simulink model "verify_Pressure_Drop_Ceta_mdl"  (R2016b)
settings: Solver=VariableStepDiscrete  StartTime=0.0  StopTime=100  MaxStep=10  RelTol=1e-3  EnableMultiTasking=on
libraries: carnot x3, simulink x1
settings Model: Creator=drhf  LastModifiedBy=drhf
settings DataIOCC: LimitDataPoints=on  SaveFormat=Array  SignalLoggingSaveFormat=ModelDataLogs
settings OptimizationCC: ExpressionDepthLimit=2147483647  LifeSpan=inf
settings DebuggingCC: UnderspecifiedInitializationDetection=Classic  MergeDetectMultiDrivingBlocksExec=none  SolverPrmCheckMsg=warning  FcnCallInpInsideContextMsg=warning  StateNameClashWarn=warning  SFUnexpectedBacktrackingDiag=warning  SFNoUnconditionalDefaultTransitionDiag=warning  SFExecutionAtInitializationDiag=none
settings HardwareCC: ProdBitPerPointer=32  ProdBitPerSizeT=32  ProdBitPerPtrDiffT=32  ProdLargestAtomicFloat=None  ProdIntDivRoundTo=Undefined  ProdEndianess=Unspecified  ProdWordSize=32  ProdHWDeviceType=32-bit Generic
settings ModelReferenceCC: PropagateSignalLabelsOutOfModel=off
settings GRTTargetCC: TargetLangStandard=C89/C90 (ANSI)  GeneratePreprocessorConditionals=Disable all  CombineOutputUpdateFcns=off  GRTInterface=on
settings ConfigComp: CovMetricSettings=dw  CovHtmlReporting=on  CovSaveCumulativeToWorkspaceVar=on  CovSaveSingleToWorkspaceVar=on  CovExternalEMLEnable=off

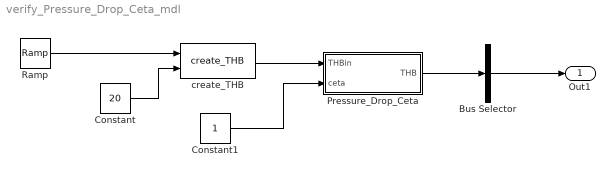
== system verify_Pressure_Drop_Ceta_mdl ==
  Bus Selector : BusSelector  OutputSignals=MassFlow,Pressure,DPConstant,DPLinear,DPQuadratic  OutputAsBus=on
  Constant : Constant  Value=20
  Constant1 : Constant
  Pressure_Drop_Ceta : Subsystem  mask(fixed pressure drop){con=101, lin=202, qua=303}
      mask prompts: con "c : constant (static) pressure drop in Pa"; lin "l : linear pressure drop Pa/(kg/s)"; qua "q : quadratic pressure drop Pa/(kg/s)²"
      mask help:
      | Constant parameters for pressure drop in a flow.
      | dp = c + l*mdot + q*mdot²
      | Calculation is done for ID > 10000 (dp = f(l, q), c is neglected) and ID > 20000 (dp = f(c,l,q)).
      | Applied directly to the THB bus.
      mask Help: web(fullfile(path_carnot('help'),'Pressure_Drop_Fix.html'),'-helpbrowser')
  Ramp : simulink/Sources/Ramp  slope=0.01  start=0  X0=0
  create_THB : carnot/Source/Simple/create_THB  p=1e5  fluid=Water  mix=0  mix2=0  mix3=0  dia=0.02  hgt=0  mID=Pressure Drop from Massflow
  Out1 : Outport
  wires:
  create_THB/1 -> Pressure_Drop_Ceta/1(THBin)
  Pressure_Drop_Ceta/1(THB) -> Bus Selector/1
  Bus Selector/1 -> Out1/1
  Ramp/1 -> create_THB/1
  Constant/1 -> create_THB/2
  Constant1/1 -> Pressure_Drop_Ceta/2(ceta)

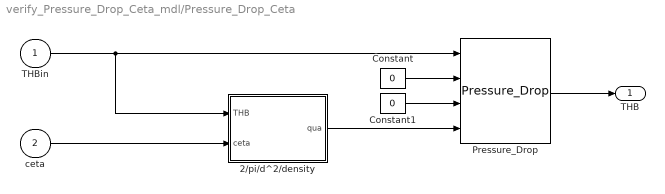
== system verify_Pressure_Drop_Ceta_mdl/Pressure_Drop_Ceta ==
  THBin : Inport
  ceta : Inport  Port=2
  2/pi/d^2/density : Subsystem
  Constant : Constant  Value=0
  Constant1 : Constant  Value=0
  Pressure_Drop : carnot/Basic/Pressure_Drop/Pressure_Drop
  THB : Outport
  wires:
  Pressure_Drop/1 -> THB/1
  THBin/1 -> 2/pi/d^2/density/1(THB), Pressure_Drop/1
  Constant/1 -> Pressure_Drop/2
  Constant1/1 -> Pressure_Drop/3
  2/pi/d^2/density/1(qua) -> Pressure_Drop/4
  ceta/1 -> 2/pi/d^2/density/2(ceta)

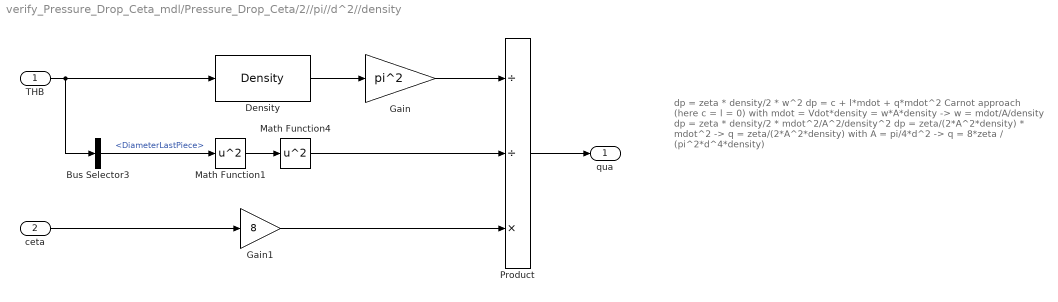
== system verify_Pressure_Drop_Ceta_mdl/Pressure_Drop_Ceta/2//pi//d^2//density ==
  note: dp = zeta * density/2 * w^2
      | dp = c + l*mdot + q*mdot^2    Carnot approach (here c = l = 0)
      | with mdot = Vdot*density = w*A*density  -> w = mdot/A/density
      | dp = zeta * density/2 * mdot^2/A^2/density^2
      | dp = zeta/(2*A^2*density) * mdot^2
      | -> q = zeta/(2*A^2*density)
      | with A = pi/4*d^2
      | -> q = 8*zeta / (pi^2*d^4*density)
  THB : Inport
  ceta : Inport  Port=2
  Bus Selector3 : BusSelector  OutputSignals=DiameterLastPiece
  Density : carnot/Basic/Material_Properties/Density  VariantControl=CarlibClassic  INPUTARGUMENTS=THB  DEBUGLEVEL=DEBUGLEVEL  MAXTOTALWARNINGS=inf  MAXCONSECUTIVEWARNINGS=inf  WRITETOFILE=0  FILENAME='errors.txt'
  Gain : Gain  Gain=pi^2
  Gain1 : Gain  Gain=8
  Math Function1 : Math  Operator=square  SaturateOnIntegerOverflow=on
  Math Function4 : Math  Operator=square  SaturateOnIntegerOverflow=on
  Product : Product  Inputs=//*  RndMeth=Zero
  qua : Outport
  wires:
  Product/1 -> qua/1
  Gain/1 -> Product/1
  THB/1 -> Density/1, Bus Selector3/1
  Density/1 -> Gain/1
  Bus Selector3/1 -> Math Function1/1  "<DiameterLastPiece>"
  Math Function1/1 -> Math Function4/1
  Math Function4/1 -> Product/2
  ceta/1 -> Gain1/1
  Gain1/1 -> Product/3
